simulink model "BiCopter_Control_V2"  (R2022a)
settings: Solver=VariableStepAuto  StartTime=0.0  StopTime=10  RelTol=1e-3
values from neighbouring files (symbols this model uses):
  At = [0 1; 0 0]    [BiCopter_V0.m]    (also in BiCopter_runner.m)
  Bt = [0;1/J]    [BiCopter_V0.m]    (also in BiCopter_runner.m)
  C = [eye(2) zeros(2)]    [BiCopter_V0.m]    (also in BiCopter_runner.m)
  C12_IL = I12([8 11],:)    [BiCopter_V0.m]    (also in BiCopter_runner.m = I12(5:6,:))
  C12_OL = I12([1 3 4 6],:)    [BiCopter_V0.m]    (also in BiCopter_runner.m = I12(1:4,:))
  Ct = [1 0]    [BiCopter_V0.m]    (also in BiCopter_runner.m)
  inertia = [m J J J]'    [BiCopter_runner.m]
  Kq = Ka(:,5:6)    [BiCopter_V0.m]    (also in BiCopter_runner.m)
  Ktq = Kta(:,3)    [BiCopter_V0.m]    (also in BiCopter_runner.m)
  Ktx = Kta(:,1:2)    [BiCopter_V0.m]    (also in BiCopter_runner.m)
  Kx = Ka(:,1:4)    [BiCopter_V0.m]    (also in BiCopter_runner.m)
  m = 2    [BiCopter_V0.m]    (also in BiCopter_runner.m)
  theta_r = rand(1,1)    [BiCopter_V0.m]    (also in BiCopter_runner.m)
  x_r = rand(2,1)    [BiCopter_V0.m]    (also in BiCopter_runner.m = randn(2,1))
settings Model: Creator=Ankit  LastModifiedBy=Ankit

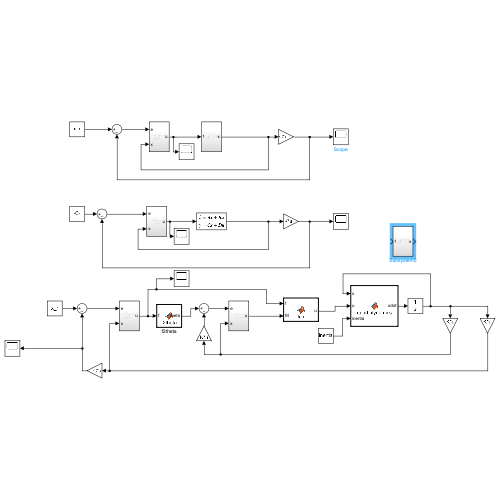
[thumbnail: Simulink's stored preview of the top-level diagram]
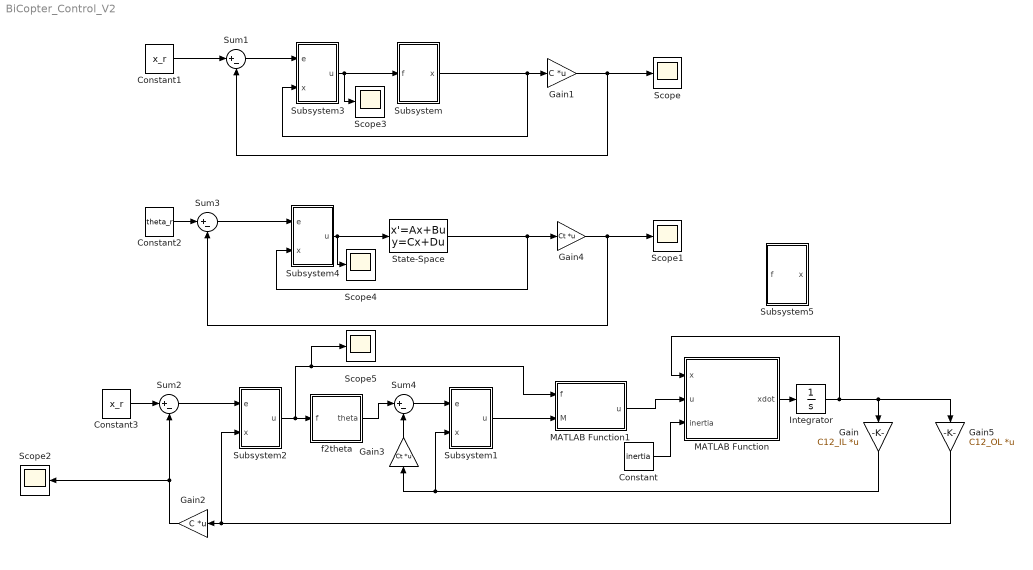
== system BiCopter_Control_V2 ==
  Constant : Constant  Value=inertia
  Constant1 : Constant  Value=x_r
  Constant2 : Constant  Value=theta_r
  Constant3 : Constant  Value=x_r
  Gain : Gain  Gain=C12_IL  Multiplication=Matrix(K*u)
  Gain1 : Gain  Gain=C  Multiplication=Matrix(K*u)
  Gain2 : Gain  Gain=C  Multiplication=Matrix(K*u)
  Gain3 : Gain  Gain=Ct  Multiplication=Matrix(K*u)
  Gain4 : Gain  Gain=Ct  Multiplication=Matrix(K*u)
  Gain5 : Gain  Gain=C12_OL  Multiplication=Matrix(K*u)
  Integrator : Integrator  InitialCondition=zeros(12,1)
  MATLAB Function : MATLAB Function  TreatAsAtomicUnit=on
  MATLAB Function1 : MATLAB Function  TreatAsAtomicUnit=on
  Scope{,1..5} (6 alike) : Scope
  State-Space : StateSpace  A=At  B=Bt  C=eye(2)  D=zeros(2,1)  InitialCondition=0
  Subsystem : Subsystem
  Subsystem1 : Subsystem
  Subsystem2 : Subsystem
  Subsystem3 : Subsystem
  Subsystem4 : Subsystem
  Subsystem5 : Subsystem
  Sum{1..4} (4 alike) : Sum  Inputs=|+-
  f2theta : MATLAB Function  TreatAsAtomicUnit=on
  wires:
  Gain1/1 -> Scope/1, Sum1/2
  Constant1/1 -> Sum1/1
  Subsystem/1(x) -> Gain1/1, Subsystem3/2(x)
  Gain4/1 -> Scope1/1, Sum3/2
  State-Space/1 -> Gain4/1, Subsystem4/2(x)
  Constant2/1 -> Sum3/1
  Sum1/1 -> Subsystem3/1(e)
  Subsystem3/1(u) -> Scope3/1, Subsystem/1(f)
  Sum3/1 -> Subsystem4/1(e)
  Subsystem4/1(u) -> Scope4/1, State-Space/1
  Sum2/1 -> Subsystem2/1(e)
  Gain2/1 -> Scope2/1, Sum2/2
  Constant3/1 -> Sum2/1
  Sum4/1 -> Subsystem1/1(e)
  Subsystem1/1(u) -> MATLAB Function1/2(M)
  Gain3/1 -> Sum4/2
  MATLAB Function/1(xdot) -> Integrator/1
  Integrator/1 -> Gain5/1, Gain/1, MATLAB Function/1(x)
  Gain/1 -> Subsystem1/2(x), Gain3/1
  Gain5/1 -> Subsystem2/2(x), Gain2/1
  f2theta/1(theta) -> Sum4/1
  Subsystem2/1(u) -> Scope5/1, MATLAB Function1/1(f), f2theta/1(f)
  MATLAB Function1/1(u) -> MATLAB Function/2(u)
  Constant/1 -> MATLAB Function/3(inertia)

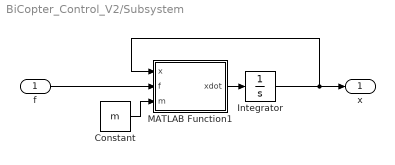
== system BiCopter_Control_V2/Subsystem ==
  f : Inport
  Constant : Constant  Value=m
  Integrator : Integrator
  MATLAB Function1 : MATLAB Function  TreatAsAtomicUnit=on
  x : Outport
  wires:
  Constant/1 -> MATLAB Function1/3(m)
  MATLAB Function1/1(xdot) -> Integrator/1
  f/1 -> MATLAB Function1/2(f)
  Integrator/1 -> MATLAB Function1/1(x), x/1

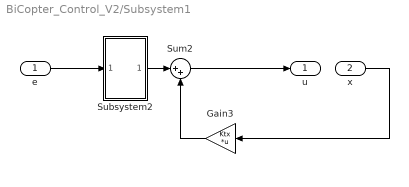
== system BiCopter_Control_V2/Subsystem1 ==
  e : Inport
  x : Inport  Port=2
  Gain3 : Gain  Gain=Ktx  Multiplication=Matrix(K*u)
  Subsystem2 : Subsystem
  Sum2 : Sum  Inputs=|++
  u : Outport
  wires:
  Subsystem2/1(Out1) -> Sum2/1
  Gain3/1 -> Sum2/2
  Sum2/1 -> u/1
  e/1 -> Subsystem2/1(In1)
  x/1 -> Gain3/1

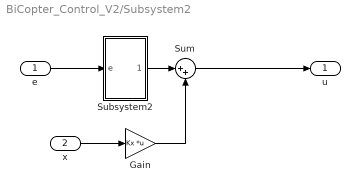
== system BiCopter_Control_V2/Subsystem2 ==
  e : Inport
  x : Inport  Port=2
  Gain : Gain  Gain=Kx  Multiplication=Matrix(K*u)
  Subsystem2 : Subsystem
  Sum : Sum  Inputs=|++
  u : Outport
  wires:
  e/1 -> Subsystem2/1(e)
  Gain/1 -> Sum/2
  Subsystem2/1(u_int) -> Sum/1
  x/1 -> Gain/1
  Sum/1 -> u/1

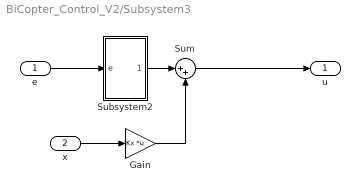
== system BiCopter_Control_V2/Subsystem3 ==
  e : Inport
  x : Inport  Port=2
  Gain : Gain  Gain=Kx  Multiplication=Matrix(K*u)
  Subsystem2 : Subsystem
  Sum : Sum  Inputs=|++
  u : Outport
  wires:
  e/1 -> Subsystem2/1(e)
  Gain/1 -> Sum/2
  Subsystem2/1(u_int) -> Sum/1
  x/1 -> Gain/1
  Sum/1 -> u/1

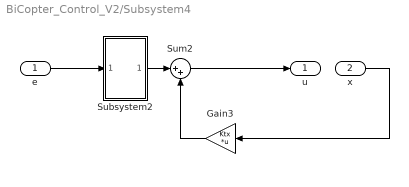
== system BiCopter_Control_V2/Subsystem4 ==
  e : Inport
  x : Inport  Port=2
  Gain3 : Gain  Gain=Ktx  Multiplication=Matrix(K*u)
  Subsystem2 : Subsystem
  Sum2 : Sum  Inputs=|++
  u : Outport
  wires:
  Subsystem2/1(Out1) -> Sum2/1
  Gain3/1 -> Sum2/2
  Sum2/1 -> u/1
  e/1 -> Subsystem2/1(In1)
  x/1 -> Gain3/1

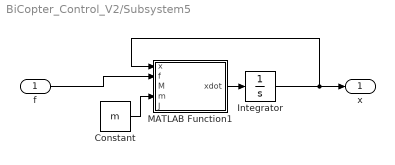
== system BiCopter_Control_V2/Subsystem5 ==
  f : Inport
  Constant : Constant  Value=m
  Integrator : Integrator
  MATLAB Function1 : MATLAB Function  TreatAsAtomicUnit=on
  x : Outport
  wires:
  Constant/1 -> MATLAB Function1/4(m)
  MATLAB Function1/1(xdot) -> Integrator/1
  f/1 -> MATLAB Function1/2(f)
  Integrator/1 -> MATLAB Function1/1(x), x/1

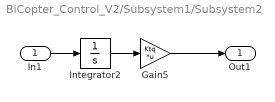
== system BiCopter_Control_V2/Subsystem1/Subsystem2 ==
  In1 : Inport
  Gain5 : Gain  Gain=Ktq  Multiplication=Matrix(K*u)
  Integrator2 : Integrator
  Out1 : Outport
  wires:
  Integrator2/1 -> Gain5/1
  Gain5/1 -> Out1/1
  In1/1 -> Integrator2/1

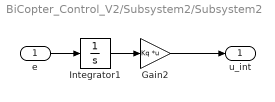
== system BiCopter_Control_V2/Subsystem2/Subsystem2 ==
  e : Inport
  Gain2 : Gain  Gain=Kq  Multiplication=Matrix(K*u)
  Integrator1 : Integrator
  u_int : Outport
  wires:
  Integrator1/1 -> Gain2/1
  Gain2/1 -> u_int/1
  e/1 -> Integrator1/1

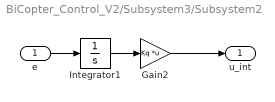
== system BiCopter_Control_V2/Subsystem3/Subsystem2 ==
  e : Inport
  Gain2 : Gain  Gain=Kq  Multiplication=Matrix(K*u)
  Integrator1 : Integrator
  u_int : Outport
  wires:
  Integrator1/1 -> Gain2/1
  Gain2/1 -> u_int/1
  e/1 -> Integrator1/1

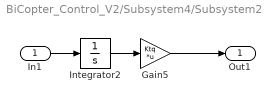
== system BiCopter_Control_V2/Subsystem4/Subsystem2 ==
  In1 : Inport
  Gain5 : Gain  Gain=Ktq  Multiplication=Matrix(K*u)
  Integrator2 : Integrator
  Out1 : Outport
  wires:
  Integrator2/1 -> Gain5/1
  Gain5/1 -> Out1/1
  In1/1 -> Integrator2/1

== matlab function BiCopter_Control_V2/Subsystem/MATLAB Function1 ==
  data: x input; xdot output; f input; m input
function xdot = fcn(x,f,m)

xdot = zeros(4,1);

xdot(1:2,1) = x(3:4,1);

xdot(3:4,1) = f/m+[0;10];

end

== matlab function BiCopter_Control_V2/MATLAB Function ==
  data: x input; u input; xdot output; inertia input
function xdot  = quad_dynamics(x,u,inertia)

m = inertia(1);
J = diag(inertia(2:4)); blkdiag(10,10,1);

r = x(1:3,1);
v = x(4:6,1);

Eul_Angles = x(7:9,1);
omega_QE = x(10:12,1);

force = u(1);
moment = u(2:4);

g = [0;0;10];

xdot = x*0;

Phi     = Eul_Angles(1);
Theta   = Eul_Angles(2);
Psi     = Eul_Angles(3);


[O3psi, O2theta, O1phi] = orientation_matrices(Phi, Theta, Psi);

xdot(1:3,1) = v;
xdot(4:6,1) = g + force/m*transpose(O3psi) * transpose(O2theta) * transpose(O1phi)*[0;0;1];

xdot(7:9,1) = S_Phi_Theta_inv(Phi,Theta)*omega_QE;
xdot(10:12,1) = J\(-cross(omega_QE,J*omega_QE)+moment);


end

function S = S_Phi_Theta_inv(Phi,Theta)
S = [1 sin(Phi)*tan(Theta) cos(Phi)*tan(Theta);
    0 cos(Phi) -sin(Phi);
    0 sin(Phi)*sec(Theta) cos(Phi)*sec(Theta)];
end

function [O3psi, O2theta, O1phi] = orientation_matrices(phi, theta, psi);
O3psi = [cos(psi) sin(psi) 0;
    -sin(psi) cos(psi) 0;
    0 0 1];
O2theta = [cos(theta) 0 -sin(theta);
    0 1 0
    sin(theta) 0 cos(theta)];
O1phi = [1 0 0
    0 cos(phi) sin(phi);
    0 -sin(phi) cos(phi) ;];
end

== matlab function BiCopter_Control_V2/f2theta ==
  data: f input; theta output
function theta = f2theta(f)

theta = atan2(-f(1),-f(2));

== matlab function BiCopter_Control_V2/MATLAB Function1 ==
  data: f input; u output; M input
function u = fcn(f, M)

u = zeros(4,1);
u(1) = norm(f);

u(2) = M;

== matlab function BiCopter_Control_V2/Subsystem5/MATLAB Function1 ==
  data: x input; xdot output; f input; M input; m input; J input
function xdot = fcn(x,f,M,m,J)

xdot = zeros(6,1);

xdot(1:2,1) = x(3:4,1);

xdot(3:4,1) = -f/m*[sin(x(5)); cos(x(5))]+[0;10];

xdot(5,1) = x(6);

xdot(6,1) = M/J;






end
